simulink model "DCmotor_modeling_statespace"  (R2015b)
settings: Solver=ode45  StartTime=0.0  StopTime=3  RelTol=1e-3
values from neighbouring files (symbols this model uses):
  A = [-R/L 0 -Ke/L ; 0 0 1 ; Kt/J 0 -Kb/J]    [DCmotor_modeling_ss.m]
  B = 0.1    [BLDCmotor_modeling_param.m]    (also in DCmotor_modeling_ss.m = [1/L; 0; 0])
  C = [0 1 0]    [DCmotor_modeling_ss.m]
  D = zeros(1,1)    [DCmotor_modeling_ss.m]
settings Model: Creator=weberhsu  LastModifiedBy=root
settings HardwareCC: ProdWordSize=32  ProdHWDeviceType=Specified

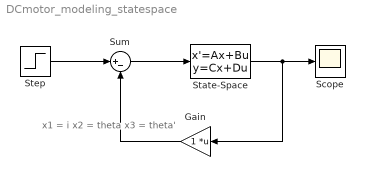
== system DCmotor_modeling_statespace ==
  note: x1 = i
      | x2 = theta
      | x3 = theta'
  Gain : Gain  Multiplication=Matrix(K*u)
  Scope : Scope
  State-Space : StateSpace  A=A  B=B  C=C  D=D  X0=0
  Step : Step  SampleTime=0
  Sum : Sum  Inputs=|+-
  wires:
  State-Space/1 -> Gain/1, Scope/1
  Step/1 -> Sum/1
  Sum/1 -> State-Space/1
  Gain/1 -> Sum/2
